simulink model "g"  (R2020a)
settings: Solver=FixedStepAuto  StartTime=0  StopTime=10.67  FixedStep=0.01  RelTol=1e-3
undefined symbols (not defined in the file): delay, VSA, VSM
settings Model: Creator=yizha  LastModifiedBy=Brock
settings DataIOCC: ReturnWorkspaceOutputs=off
settings DebuggingCC: ArithmeticOperatorsInVariantConditions=warning
settings SFSimCC: CustomCodeUndefinedFunction=UseInterfaceOnly

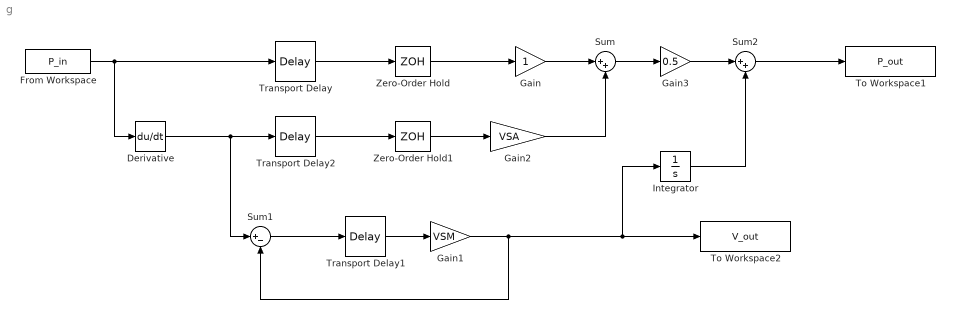
== system g ==
  Derivative : Derivative
  From Workspace : FromWorkspace  VariableName=P_in
  Gain : Gain
  Gain1 : Gain  Gain=VSM
  Gain2 : Gain  Gain=VSA
  Gain3 : Gain  Gain=0.5
  Integrator : Integrator
  Sum : Sum  Inputs=|++
  Sum1 : Sum  Inputs=|+-
  Sum2 : Sum  Inputs=|++
  To Workspace1 : ToWorkspace  VariableName=P_out  SampleTime=-1
  To Workspace2 : ToWorkspace  VariableName=V_out  SampleTime=-1
  Transport Delay : TransportDelay  DelayTime=delay
  Transport Delay1 : TransportDelay  DelayTime=delay
  Transport Delay2 : TransportDelay  DelayTime=delay
  Zero-Order Hold : ZeroOrderHold  SampleTime=delay
  Zero-Order Hold1 : ZeroOrderHold  SampleTime=delay
  wires:
  Sum1/1 -> Transport Delay1/1
  Transport Delay1/1 -> Gain1/1
  Derivative/1 -> Sum1/1, Transport Delay2/1
  Transport Delay/1 -> Zero-Order Hold/1
  Gain/1 -> Sum/1
  Zero-Order Hold1/1 -> Gain2/1
  From Workspace/1 -> Derivative/1, Transport Delay/1
  Zero-Order Hold/1 -> Gain/1
  Transport Delay2/1 -> Zero-Order Hold1/1
  Gain2/1 -> Sum/2
  Sum2/1 -> To Workspace1/1
  Integrator/1 -> Sum2/2
  Sum/1 -> Gain3/1
  Gain3/1 -> Sum2/1
  Gain1/1 -> To Workspace2/1, Integrator/1, Sum1/2
